simulink model "fuelCycle_w_trapping"  (R2023b)
settings: Solver=ode15s  StartTime=0.0  StopTime=sim_time  MinStep=1e-4  RelTol=1e-4
values from neighbouring files (symbols this model uses):
  AF = 90    [BOTH_scenario_inputData.m]    (also in FC_scenario_inputData.m; PO_scenario_inputData.m = 0.7; inputData.m = 70; parametric_analysis_AF.m = AF_array(i))
  eta2 = 0.95    [BOTH_scenario_inputData.m]    (also in FC_scenario_inputData.m; PO_scenario_inputData.m; inputData.m; parametric_analysis_eta_tes.m = eta_tes_array(i))
  f51 = 0.33    [BOTH_scenario_inputData.m]    (also in FC_scenario_inputData.m; PO_scenario_inputData.m; inputData.m; worst_case_InputData.m)
  f53 = 0.33    [BOTH_scenario_inputData.m]    (also in FC_scenario_inputData.m; PO_scenario_inputData.m; inputData.m; worst_case_InputData.m)
  f54 = 1 - f51 - f53 - f56    (= 0.3399)    [BOTH_scenario_inputData.m]    (also in FC_scenario_inputData.m; PO_scenario_inputData.m; inputData.m; worst_case_InputData.m)
  f96 = 0.1    [BOTH_scenario_inputData.m]    (also in FC_scenario_inputData.m; PO_scenario_inputData.m; inputData.m; worst_case_InputData.m)
  f_dir = 0.7    [BOTH_scenario_inputData.m]    (also in FC_scenario_inputData.m; PO_scenario_inputData.m = 0.3; inputData.m = 0.3; parametric_analysis_f_dir.m = f_dir_array(i))
  f_permanent_trap = 0    [inputData_trapping.m]    (also in parametric_analysis_trapping.m = f_permanent_trap_array(i))
  f_permanent_trap_structural = 0    [inputData_trapping.m]
  fp3 = 1e-4    (= 0.0001)    [BOTH_scenario_inputData.m]    (also in FC_scenario_inputData.m; PO_scenario_inputData.m; inputData.m; parametric_analysis_f_p.m = f_p(i) / 2)
  fp4 = 1e-4    (= 0.0001)    [BOTH_scenario_inputData.m]    (also in FC_scenario_inputData.m; PO_scenario_inputData.m; inputData.m; parametric_analysis_f_p.m = f_p(i) / 2)
  I_s_0 = 1.4    [fuelCycleSimulator.m]    (also in parametric_analysis_AF.m = 0.8; parametric_analysis_epsi.m = 0.8; parametric_analysis_eta_tes.m = 0.8; parametric_analysis_f_dir.m = 0.8)
  lambda = 1.73e-9    (= 1.73e-09)    [BOTH_scenario_inputData.m]    (also in FC_scenario_inputData.m; PO_scenario_inputData.m; inputData.m; inputData_trapping.m = a_tungsten/2/sqrt(2))
  m_u = 1.6e-27    [inputData_trapping-lap-meschini.m]    (also in inputData_trapping.m)
  N_dot = 8.99e-7    (= 8.99e-07)    [BOTH_scenario_inputData.m]    (also in FC_scenario_inputData.m = 9.3e-07; PO_scenario_inputData.m = 9.3e-07; inputData.m = 9.3e-07; worst_case_InputData.m = 9.3e-07)
  n_structural = (rho_structural*1e3) / PM_structural * N_a    (= 7.36894684052e+25)    [inputData_trapping-lap-meschini.m]    (also in inputData_trapping.m = 2.57913139418e+29)
  n_trap = 1e-4    (= 0.0001)    [inputData_trapping.m]    (also in parametric_analysis_trapping.m = n_trap_array(j))
  n_trap_structural = n_trap_vcrti    (= 0.0001)    [inputData_trapping-lap-meschini.m]    (also in inputData_trapping.m; parametric_analysis_trapping.m = n_trap_array(j))
  n_tungsten = (rho_tungsten*1e3) / PM_tungsten * N_a    (= 6.32342763874e+25)    [inputData_trapping-lap-meschini.m]    (also in inputData_trapping.m = 2.21319967356e+28)
  T1 = 1/((1 + epsi)/tau1 + lambda)    [BOTH_scenario_inputData.m]    (also in FC_scenario_inputData.m; PO_scenario_inputData.m; inputData.m; parametric_analysis_epsi.m)
  T12 = 1/((1 + epsi)/tau12 + lambda)    [BOTH_scenario_inputData.m]    (also in FC_scenario_inputData.m; PO_scenario_inputData.m; inputData.m; parametric_analysis_epsi.m)
  T2 = 1/((1 + epsi)/tau2 + lambda)    [BOTH_scenario_inputData.m]    (also in FC_scenario_inputData.m; PO_scenario_inputData.m; inputData.m; parametric_analysis_epsi.m)
  T3 = 1/((1 + 0)/tau3 + lambda)    [BOTH_scenario_inputData.m]    (also in FC_scenario_inputData.m; PO_scenario_inputData.m; inputData.m; parametric_analysis_epsi.m)
  T4 = 1/((1 + 0)/tau4 + lambda)    [BOTH_scenario_inputData.m]    (also in FC_scenario_inputData.m; PO_scenario_inputData.m; inputData.m; parametric_analysis_epsi.m)
  T7 = 1/((1 + epsi)/tau7 + lambda)    [BOTH_scenario_inputData.m]    (also in FC_scenario_inputData.m; PO_scenario_inputData.m; inputData.m; parametric_analysis_epsi.m)
  T8 = 1/((1 + epsi)/tau8 + lambda)    [BOTH_scenario_inputData.m]    (also in FC_scenario_inputData.m; PO_scenario_inputData.m; inputData.m; parametric_analysis_TBE.m)
  T9 = 1/((1 + epsi)/tau9 + lambda)    [BOTH_scenario_inputData.m]    (also in FC_scenario_inputData.m; PO_scenario_inputData.m; inputData.m; parametric_analysis_TBE.m)
  T_replacement = 100*8760*3600    (= 3153600000)    [inputData.m]
  tau1 = 1.25*3600    (= 4500)    [BOTH_scenario_inputData.m]    (also in FC_scenario_inputData.m; PO_scenario_inputData.m; inputData.m; parametric_analysis_t_blanket.m = tau1_array(i))
  tau12 = 100    [BOTH_scenario_inputData.m]    (also in FC_scenario_inputData.m; PO_scenario_inputData.m; inputData.m; worst_case_InputData.m)
  tau2 = 1*24*3600    (= 86400)    [BOTH_scenario_inputData.m]    (also in FC_scenario_inputData.m; PO_scenario_inputData.m; inputData.m; worst_case_InputData.m)
  tau3 = 1000    [BOTH_scenario_inputData.m]    (also in FC_scenario_inputData.m; PO_scenario_inputData.m; inputData.m; worst_case_InputData.m)
  tau4 = 1000    [BOTH_scenario_inputData.m]    (also in FC_scenario_inputData.m; PO_scenario_inputData.m; inputData.m; worst_case_InputData.m)
  tau5 = 1000    [BOTH_scenario_inputData.m]    (also in FC_scenario_inputData.m; PO_scenario_inputData.m; inputData.m; worst_case_InputData.m)
  tau6 = 3600    [BOTH_scenario_inputData.m]    (also in FC_scenario_inputData.m; PO_scenario_inputData.m; inputData.m; worst_case_InputData.m)
  tau7 = 600    [BOTH_scenario_inputData.m]    (also in FC_scenario_inputData.m; PO_scenario_inputData.m; inputData.m; worst_case_InputData.m)
  tau8 = 0.1*3600    (= 360)    [BOTH_scenario_inputData.m]    (also in FC_scenario_inputData.m; PO_scenario_inputData.m; inputData.m = 3600; parametric_analysis_TBE.m = t_p*0.1)
  tau9 = 0.9*3600    (= 3240)    [BOTH_scenario_inputData.m]    (also in FC_scenario_inputData.m; PO_scenario_inputData.m = 14040; inputData.m = 10800; parametric_analysis_TBE.m = t_p*0.9)
  tau_detrap = 1 / nu_detrap* relaxation_coefficient    [inputData_trapping.m]
  tau_detrap_structural = 1 / nu_detrap_structural* relaxation_coefficient    [inputData_trapping-lap-meschini.m]    (also in inputData_trapping.m)
  tau_permanent = 100 * 24 *3600    (= 8640000)    [inputData_trapping.m]
  tau_permanent_structural = 100 * 24 *3600    (= 8640000)    [inputData_trapping.m]
  TBE = 0.1    [BOTH_scenario_inputData.m]    (also in FC_scenario_inputData.m = 0.02; PO_scenario_inputData.m; inputData.m = 0.02; parametric_analysis_AF.m = TBE_array(j))
  TBR = 1.06    [fuelCycleSimulator.m]    (also in parametric_analysis_AF.m = 1; parametric_analysis_TBE.m = 1; parametric_analysis_epsi.m = 1; parametric_analysis_eta_tes.m = 1)
  V_structural = 3.5e6    (= 3500000)    [inputData_trapping-lap-meschini.m]    (also in inputData_trapping.m)
  V_tungsten = 0.35e6    (= 350000)    [inputData_trapping-lap-meschini.m]    (also in inputData_trapping.m)
libraries: arc x4
settings Model: SimulationMode=accelerator  Creator=smesc  LastModifiedBy=smesc
settings SolverCC: InitialStep=1e-4  MaxConsecutiveMinStep=10  ShapePreserveControl=EnableAll  ZeroCrossAlgorithm=Adaptive
settings OptimizationCC: ReuseModelBlockBuffer=off
settings ModelReferenceCC: EnableRefExpFcnMdlSchedulingChecks=on

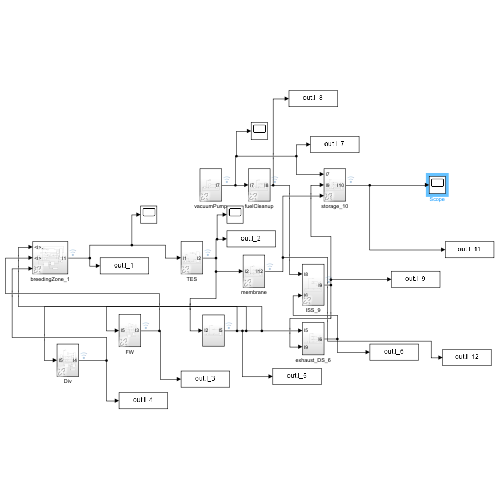
[thumbnail: Simulink's stored preview of the top-level diagram]
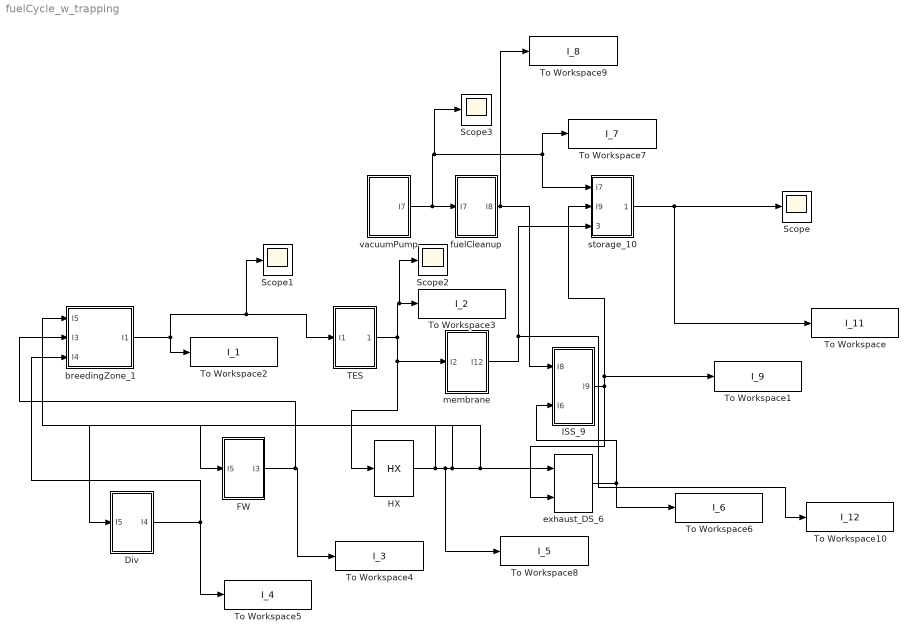
== system fuelCycle_w_trapping ==
  Div : Subsystem  AncestorBlock=arc/divertor_4
      settings: LibrarySourceBlock=arc/divertor_4
  FW : Subsystem  AncestorBlock=arc/FW_3
      settings: LibrarySourceBlock=arc/FW_3
  HX : arc/HX  Tag=HX  SystemSampleTime=-1  VariantActivationTime=update diagram  AllowFlexibleInterface=on  Latency=0  AutoFrameSizeCalculation=off
  ISS_9 : Subsystem  AncestorBlock=arc/ISS_9
      settings: LibrarySourceBlock=arc/ISS_9
  Scope{,1..3} (4 alike) : Scope
  TES : Subsystem  AncestorBlock=arc/TES_2
      settings: LibrarySourceBlock=arc/TES_2
  To Workspace : ToWorkspace  VariableName=I_11  SampleTime=-1
  To Workspace1 : ToWorkspace  VariableName=I_9  SampleTime=-1
  To Workspace10 : ToWorkspace  VariableName=I_12  SampleTime=-1
  To Workspace2 : ToWorkspace  VariableName=I_1  SampleTime=-1
  To Workspace3 : ToWorkspace  VariableName=I_2  SampleTime=-1
  To Workspace4 : ToWorkspace  VariableName=I_3  SampleTime=-1
  To Workspace5 : ToWorkspace  VariableName=I_4  SampleTime=-1
  To Workspace6 : ToWorkspace  VariableName=I_6  SampleTime=-1
  To Workspace7 : ToWorkspace  VariableName=I_7  SampleTime=-1
  To Workspace8 : ToWorkspace  VariableName=I_5  SampleTime=-1
  To Workspace9 : ToWorkspace  VariableName=I_8  SampleTime=-1
  breedingZone_1 : Subsystem  AncestorBlock=arc/breedingZone_1
      settings: LibrarySourceBlock=arc/breedingZone_1
  exhaust_DS_6 : arc/exhaust_DS  SystemSampleTime=-1  VariantActivationTime=update diagram  AllowFlexibleInterface=on  Latency=0  AutoFrameSizeCalculation=off
      link override Gain: Gain=f56/tau5
  fuelCleanup : Subsystem  AncestorBlock=arc/fuelCleanUp
  membrane : Subsystem  AncestorBlock=arc/fuelCleanUp_8
      settings: LibrarySourceBlock=arc/fuelCleanUp_8
  storage_10 : Subsystem  AncestorBlock=arc/storage_10
      settings: LibrarySourceBlock=arc/storage_10
  vacuumPump : Subsystem  AncestorBlock=arc/pump_7
      settings: LibrarySourceBlock=arc/pump_7
  wires:
  breedingZone_1/1(I1) -> Scope1/1, TES/1(I1), To Workspace2/1
  storage_10/1(I10) -> To Workspace/1, Scope/1
  FW/1(I3) -> breedingZone_1/2(I3), To Workspace4/1
  Div/1(I4) -> breedingZone_1/3(I4), To Workspace5/1
  membrane/1(I12) -> To Workspace10/1, storage_10/3(I12)
  fuelCleanup/1(I8) -> To Workspace9/1, ISS_9/1(I8)
  vacuumPump/1(I7) -> Scope3/1, To Workspace7/1, storage_10/1(I7), fuelCleanup/1(I7)
  exhaust_DS_6/1 -> ISS_9/2(I6), To Workspace6/1
  ISS_9/1(I9) -> exhaust_DS_6/2, storage_10/2(I9), To Workspace1/1
  HX/1 -> FW/1(I5), To Workspace8/1, Div/1(I5), exhaust_DS_6/1, breedingZone_1/1(I5)
  TES/1(Output) -> Scope2/1, To Workspace3/1, membrane/1(I2), HX/1

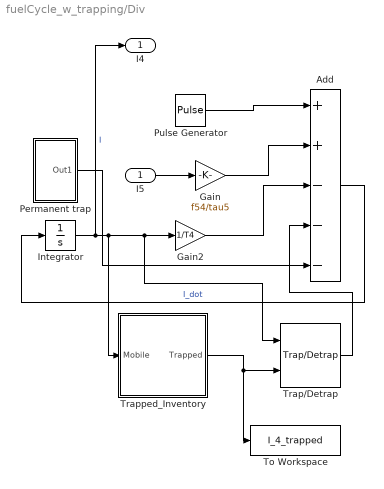
== system fuelCycle_w_trapping/Div ==
  I5 : Inport
  Add : Sum  Inputs=++---
  Gain : Gain  Gain=f54/tau5
  Gain2 : Gain  Gain=1/T4
  Integrator : Integrator
  Permanent trap : Subsystem
  Pulse Generator : DiscretePulseGenerator  PulseType=Time based  Amplitude=fp4*N_dot/TBE  Period=1800  PulseWidth=AF
  To Workspace : ToWorkspace  VariableName=I_4_trapped  SampleTime=-1
  Trap/Detrap : arc/Trap//Detrap  SystemSampleTime=-1  VariantActivationTime=update diagram  AllowFlexibleInterface=on  Latency=0  AutoFrameSizeCalculation=off
  Trapped_Inventory : Subsystem  AncestorBlock=arc/Trapped_Inventory
  I4 : Outport
  wires:
  Pulse Generator/1 -> Add/1
  Gain/1 -> Add/2
  Integrator/1 -> Trapped_Inventory/1(Mobile), Trap/Detrap/1, Gain2/1, I4/1  "I"
  Add/1 -> Integrator/1  "I_dot"
  Gain2/1 -> Add/3
  I5/1 -> Gain/1
  Trapped_Inventory/1(Trapped) -> To Workspace/1, Trap/Detrap/2
  Trap/Detrap/1 -> Add/4
  Permanent trap/1(Out1) -> Add/5

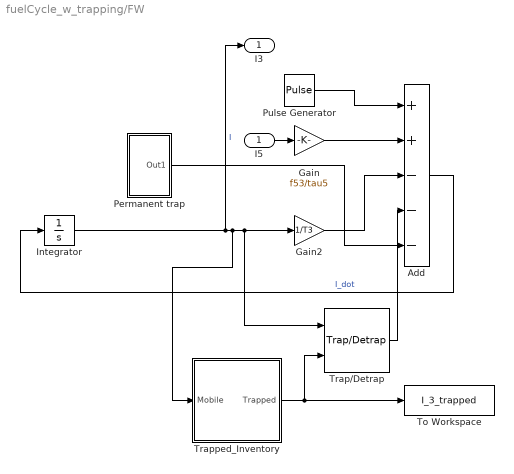
== system fuelCycle_w_trapping/FW ==
  I5 : Inport
  Add : Sum  Inputs=++---
  Gain : Gain  Gain=f53/tau5
  Gain2 : Gain  Gain=1/T3
  Integrator : Integrator
  Permanent trap : Subsystem
  Pulse Generator : DiscretePulseGenerator  PulseType=Time based  Amplitude=fp3*N_dot/TBE  Period=1800  PulseWidth=AF
  To Workspace : ToWorkspace  VariableName=I_3_trapped  SampleTime=-1
  Trap/Detrap : arc/Trap//Detrap  SystemSampleTime=-1  VariantActivationTime=update diagram  AllowFlexibleInterface=on  Latency=0  AutoFrameSizeCalculation=off
  Trapped_Inventory : Subsystem  AncestorBlock=arc/Trapped_Inventory
  I3 : Outport
  wires:
  Gain2/1 -> Add/3
  Pulse Generator/1 -> Add/1
  Integrator/1 -> I3/1, Trapped_Inventory/1(Mobile), Trap/Detrap/1, Gain2/1  "I"
  Add/1 -> Integrator/1  "I_dot"
  Gain/1 -> Add/2
  I5/1 -> Gain/1
  Trap/Detrap/1 -> Add/4
  Trapped_Inventory/1(Trapped) -> Trap/Detrap/2, To Workspace/1
  Permanent trap/1(Out1) -> Add/5

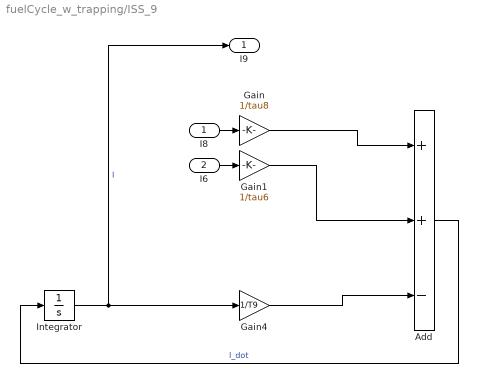
== system fuelCycle_w_trapping/ISS_9 ==
  I8 : Inport
  I6 : Inport  Port=2
  Add : Sum  Inputs=++-
  Gain : Gain  Gain=1/tau8
  Gain1 : Gain  Gain=1/tau6
  Gain4 : Gain  Gain=1/T9
  Integrator : Integrator
  I9 : Outport
  wires:
  I8/1 -> Gain/1
  Gain1/1 -> Add/2
  I6/1 -> Gain1/1
  Add/1 -> Integrator/1  "I_dot"
  Integrator/1 -> Gain4/1, I9/1  "I"
  Gain/1 -> Add/1
  Gain4/1 -> Add/3

== system fuelCycle_w_trapping/TES ==
  I1 : Inport
  Add : Sum  Inputs=+-
  Gain : Gain  Gain=1/T2
  Gain1 : Gain  Gain=1/tau1
  Integrator : Integrator
  Output : Outport
  wires:
  Gain/1 -> Add/2
  I1/1 -> Gain1/1
  Gain1/1 -> Add/1
  Integrator/1 -> Gain/1, Output/1  "I2"
  Add/1 -> Integrator/1  "I_dot"

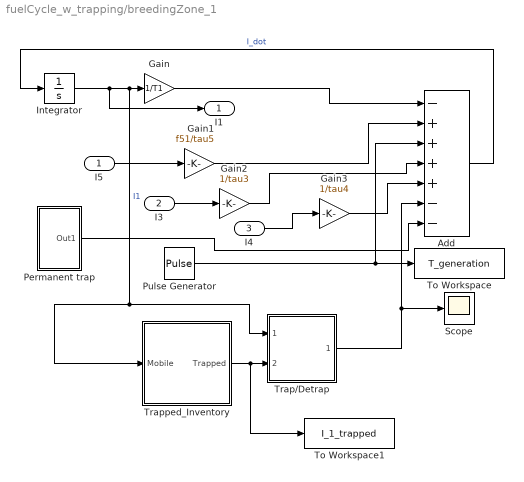
== system fuelCycle_w_trapping/breedingZone_1 ==
  I5 : Inport
  I3 : Inport  Port=2
  I4 : Inport  Port=3
  Add : Sum  Inputs=-++++--
  Gain : Gain  Gain=1/T1
  Gain1 : Gain  Gain=f51/tau5
  Gain2 : Gain  Gain=1/tau3
  Gain3 : Gain  Gain=1/tau4
  Integrator : Integrator
  Permanent trap : Subsystem
  Pulse Generator : DiscretePulseGenerator  PulseType=Time based  Amplitude=N_dot * TBR  Period=1800  PulseWidth=AF
  Scope : Scope
  To Workspace : ToWorkspace  VariableName=T_generation  SaveFormat=Timeseries  SampleTime=-1
  To Workspace1 : ToWorkspace  VariableName=I_1_trapped  SampleTime=-1
  Trap/Detrap : Subsystem  AncestorBlock=arc/Trap//Detrap
  Trapped_Inventory : Subsystem  AncestorBlock=arc/Trapped_Inventory
  I1 : Outport
  wires:
  Add/1 -> Integrator/1  "I_dot"
  Gain1/1 -> Add/2
  Integrator/1 -> Trapped_Inventory/1(Mobile), Trap/Detrap/1(Mobile), Gain/1, I1/1  "I1"
  Gain/1 -> Add/1
  I5/1 -> Gain1/1
  Pulse Generator/1 -> Add/3, To Workspace/1
  I3/1 -> Gain2/1
  Gain2/1 -> Add/4
  I4/1 -> Gain3/1
  Gain3/1 -> Add/5
  Trapped_Inventory/1(Trapped) -> To Workspace1/1, Trap/Detrap/2(Trapped)
  Trap/Detrap/1(trap_detrap) -> Scope/1, Add/6
  Permanent trap/1(Out1) -> Add/7

== system fuelCycle_w_trapping/fuelCleanup ==
  I7 : Inport
  Add : Sum  Inputs=+-
  Gain : Gain  Gain=(1-f_dir)/tau7
  Gain1 : Gain  Gain=1/T8
  Integrator : Integrator
  I8 : Outport
  wires:
  I7/1 -> Gain/1
  Gain1/1 -> Add/2
  Add/1 -> Integrator/1  "I_dot"
  Integrator/1 -> Gain1/1, I8/1  "I"
  Gain/1 -> Add/1

== system fuelCycle_w_trapping/membrane ==
  I2 : Inport
  Add : Sum  Inputs=+-
  Gain : Gain  Gain=eta2/tau2
  Gain1 : Gain  Gain=1/T12
  Integrator : Integrator
  I12 : Outport
  wires:
  I2/1 -> Gain/1
  Gain1/1 -> Add/2
  Add/1 -> Integrator/1  "I_dot"
  Integrator/1 -> Gain1/1, I12/1  "I"
  Gain/1 -> Add/1

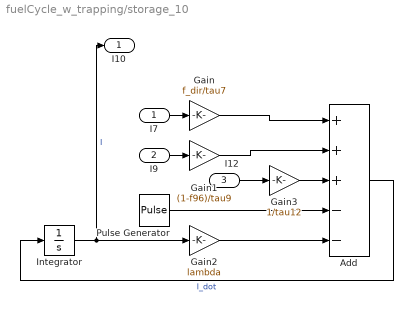
== system fuelCycle_w_trapping/storage_10 ==
  I7 : Inport
  I9 : Inport  Port=2
  I12 : Inport  Port=3
  Add : Sum  Inputs=+++--
  Gain : Gain  Gain=f_dir/tau7
  Gain1 : Gain  Gain=(1-f96)/tau9
  Gain2 : Gain  Gain=lambda
  Gain3 : Gain  Gain=1/tau12
  Integrator : Integrator  InitialCondition=I_s_0
  Pulse Generator : DiscretePulseGenerator  PulseType=Time based  Amplitude=N_dot/TBE  Period=1800  PulseWidth=AF
  I10 : Outport
  wires:
  Integrator/1 -> Gain2/1, I10/1  "I"
  I9/1 -> Gain1/1
  Gain2/1 -> Add/5
  I7/1 -> Gain/1
  Gain1/1 -> Add/2
  Gain/1 -> Add/1
  Pulse Generator/1 -> Add/4
  I12/1 -> Gain3/1
  Gain3/1 -> Add/3
  Add/1 -> Integrator/1  "I_dot"

== system fuelCycle_w_trapping/vacuumPump ==
  Add : Sum  Inputs=+-
  Gain : Gain  Gain=1/T7
  Integrator : Integrator
  Pulse Generator : DiscretePulseGenerator  PulseType=Time based  Amplitude=(1-TBE-fp3-fp4)*N_dot/TBE  Period=1800  PulseWidth=AF
  I7 : Outport
  wires:
  Gain/1 -> Add/2
  Integrator/1 -> Gain/1, I7/1  "I7"
  Pulse Generator/1 -> Add/1
  Add/1 -> Integrator/1  "I_dot"

== system fuelCycle_w_trapping/Div/Permanent trap ==
  Clock : Clock
  Exp : Math
  Gain1 : Gain  Gain=-1/tau_permanent
  Gain3 : Gain  Gain=f_permanent_trap*n_trap*n_tungsten*3*m_u*1*(V_tungsten/2)
  Scope : Scope
  Out1 : Outport
  wires:
  Gain3/1 -> Scope/1, Out1/1
  Clock/1 -> Gain1/1
  Gain1/1 -> Exp/1
  Exp/1 -> Gain3/1

== system fuelCycle_w_trapping/Div/Trapped_Inventory ==
  Mobile : Inport
  Integrator1 : Integrator
  Trap/Detrap : Subsystem
  Trapped : Outport
  wires:
  Trap/Detrap/1(Out1) -> Integrator1/1
  Mobile/1 -> Trap/Detrap/1(In1)
  Integrator1/1 -> Trap/Detrap/2(In2), Trapped/1

== system fuelCycle_w_trapping/FW/Permanent trap ==
  Clock : Clock
  Exp : Math
  Gain1 : Gain  Gain=-1/tau_permanent
  Gain3 : Gain  Gain=f_permanent_trap*n_trap*n_tungsten*3*m_u*1*(V_tungsten/2)
  Scope : Scope
  Out1 : Outport
  wires:
  Gain3/1 -> Scope/1, Out1/1
  Clock/1 -> Gain1/1
  Gain1/1 -> Exp/1
  Exp/1 -> Gain3/1

== system fuelCycle_w_trapping/FW/Trapped_Inventory ==
  Mobile : Inport
  Integrator1 : Integrator
  Trap/Detrap : Subsystem
  Trapped : Outport
  wires:
  Trap/Detrap/1(Out1) -> Integrator1/1
  Mobile/1 -> Trap/Detrap/1(In1)
  Integrator1/1 -> Trap/Detrap/2(In2), Trapped/1

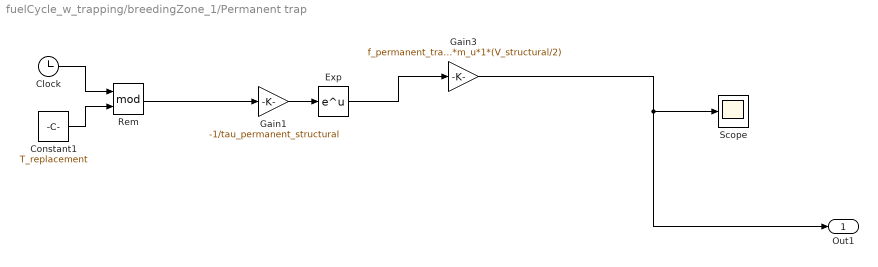
== system fuelCycle_w_trapping/breedingZone_1/Permanent trap ==
  Clock : Clock
  Constant1 : Constant  Value=T_replacement
  Exp : Math
  Gain1 : Gain  Gain=-1/tau_permanent_structural
  Gain3 : Gain  Gain=f_permanent_trap_structural*n_trap_structural*n_structural*3*m_u*1*(V_structural/2)
  Rem : Math  Operator=mod
  Scope : Scope
  Out1 : Outport
  wires:
  Gain3/1 -> Scope/1, Out1/1
  Gain1/1 -> Exp/1
  Exp/1 -> Gain3/1
  Clock/1 -> Rem/1
  Constant1/1 -> Rem/2
  Rem/1 -> Gain1/1

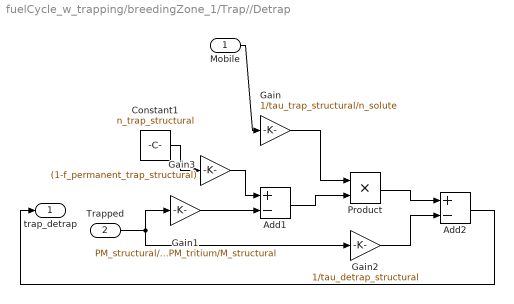
== system fuelCycle_w_trapping/breedingZone_1/Trap//Detrap ==
  Mobile : Inport
  Trapped : Inport  Port=2
  Add1 : Sum  Inputs=+-
  Add2 : Sum  Inputs=+-
  Constant1 : Constant  Value=n_trap_structural
  Gain : Gain  Gain=1/tau_trap_structural/n_solute
  Gain1 : Gain  Gain=PM_structural/PM_tritium/M_structural
  Gain2 : Gain  Gain=1/tau_detrap_structural
  Gain3 : Gain  Gain=(1-f_permanent_trap_structural)
  Product : Product
  trap_detrap : Outport
  wires:
  Trapped/1 -> Gain1/1, Gain2/1
  Gain1/1 -> Add1/2
  Add1/1 -> Product/2
  Gain2/1 -> Add2/2
  Gain/1 -> Product/1
  Mobile/1 -> Gain/1
  Add2/1 -> trap_detrap/1
  Product/1 -> Add2/1
  Constant1/1 -> Gain3/1
  Gain3/1 -> Add1/1

== system fuelCycle_w_trapping/breedingZone_1/Trapped_Inventory ==
  Mobile : Inport
  Clock : Clock
  Constant1 : Constant  Value=T_replacement
  Integrator1 : Integrator  ExternalReset=falling
  Rem : Math  Operator=mod
  Trap/Detrap : Subsystem
  Trapped : Outport
  wires:
  Trap/Detrap/1(Out1) -> Integrator1/1
  Mobile/1 -> Trap/Detrap/1(In1)
  Integrator1/1 -> Trap/Detrap/2(In2), Trapped/1
  Clock/1 -> Rem/1
  Rem/1 -> Integrator1/2
  Constant1/1 -> Rem/2

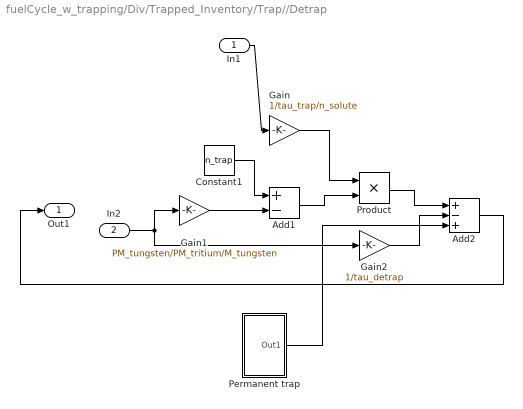
== system fuelCycle_w_trapping/Div/Trapped_Inventory/Trap//Detrap ==
  In1 : Inport
  In2 : Inport  Port=2
  Add1 : Sum  Inputs=+-
  Add2 : Sum  Inputs=+-+
  Constant1 : Constant  Value=n_trap
  Gain : Gain  Gain=1/tau_trap/n_solute
  Gain1 : Gain  Gain=PM_tungsten/PM_tritium/M_tungsten
  Gain2 : Gain  Gain=1/tau_detrap
  Permanent trap : Subsystem
  Product : Product
  Out1 : Outport
  wires:
  In2/1 -> Gain1/1, Gain2/1
  Gain1/1 -> Add1/2
  Add1/1 -> Product/2
  Gain2/1 -> Add2/2
  Constant1/1 -> Add1/1
  Gain/1 -> Product/1
  In1/1 -> Gain/1
  Add2/1 -> Out1/1
  Product/1 -> Add2/1
  Permanent trap/1(Out1) -> Add2/3

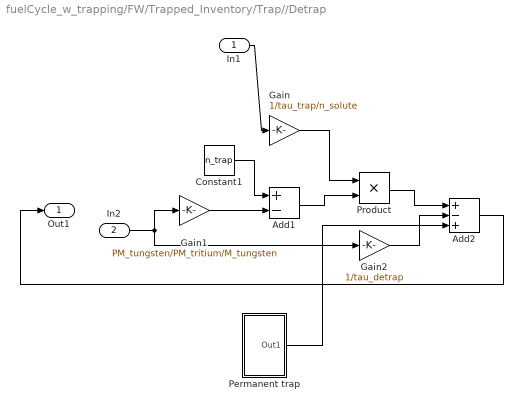
== system fuelCycle_w_trapping/FW/Trapped_Inventory/Trap//Detrap ==
  In1 : Inport
  In2 : Inport  Port=2
  Add1 : Sum  Inputs=+-
  Add2 : Sum  Inputs=+-+
  Constant1 : Constant  Value=n_trap
  Gain : Gain  Gain=1/tau_trap/n_solute
  Gain1 : Gain  Gain=PM_tungsten/PM_tritium/M_tungsten
  Gain2 : Gain  Gain=1/tau_detrap
  Permanent trap : Subsystem
  Product : Product
  Out1 : Outport
  wires:
  In2/1 -> Gain1/1, Gain2/1
  Gain1/1 -> Add1/2
  Add1/1 -> Product/2
  Gain2/1 -> Add2/2
  Constant1/1 -> Add1/1
  Gain/1 -> Product/1
  In1/1 -> Gain/1
  Add2/1 -> Out1/1
  Product/1 -> Add2/1
  Permanent trap/1(Out1) -> Add2/3

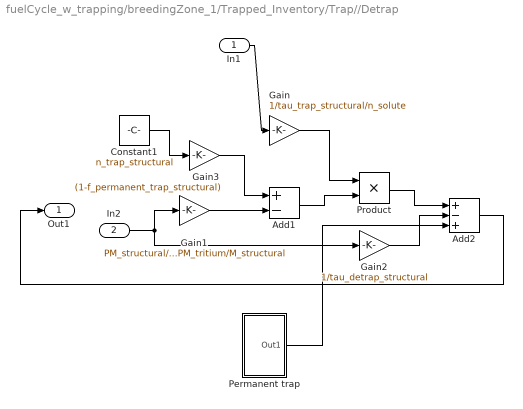
== system fuelCycle_w_trapping/breedingZone_1/Trapped_Inventory/Trap//Detrap ==
  In1 : Inport
  In2 : Inport  Port=2
  Add1 : Sum  Inputs=+-
  Add2 : Sum  Inputs=+-+
  Constant1 : Constant  Value=n_trap_structural
  Gain : Gain  Gain=1/tau_trap_structural/n_solute
  Gain1 : Gain  Gain=PM_structural/PM_tritium/M_structural
  Gain2 : Gain  Gain=1/tau_detrap_structural
  Gain3 : Gain  Gain=(1-f_permanent_trap_structural)
  Permanent trap : Subsystem
  Product : Product
  Out1 : Outport
  wires:
  In2/1 -> Gain1/1, Gain2/1
  Gain1/1 -> Add1/2
  Add1/1 -> Product/2
  Gain2/1 -> Add2/2
  Gain/1 -> Product/1
  In1/1 -> Gain/1
  Add2/1 -> Out1/1
  Product/1 -> Add2/1
  Permanent trap/1(Out1) -> Add2/3
  Constant1/1 -> Gain3/1
  Gain3/1 -> Add1/1

== system fuelCycle_w_trapping/Div/Trapped_Inventory/Trap//Detrap/Permanent trap ==
  Clock : Clock
  Exp : Math
  Gain1 : Gain  Gain=-1/tau_permanent
  Gain3 : Gain  Gain=f_permanent_trap*n_trap*n_tungsten*3*m_u*1*(V_tungsten/2)
  Scope : Scope
  Out1 : Outport
  wires:
  Gain3/1 -> Scope/1, Out1/1
  Clock/1 -> Gain1/1
  Gain1/1 -> Exp/1
  Exp/1 -> Gain3/1

== system fuelCycle_w_trapping/FW/Trapped_Inventory/Trap//Detrap/Permanent trap ==
  Clock : Clock
  Exp : Math
  Gain1 : Gain  Gain=-1/tau_permanent
  Gain3 : Gain  Gain=f_permanent_trap*n_trap*n_tungsten*3*m_u*1*(V_tungsten/2)
  Scope : Scope
  Out1 : Outport
  wires:
  Gain3/1 -> Scope/1, Out1/1
  Clock/1 -> Gain1/1
  Gain1/1 -> Exp/1
  Exp/1 -> Gain3/1

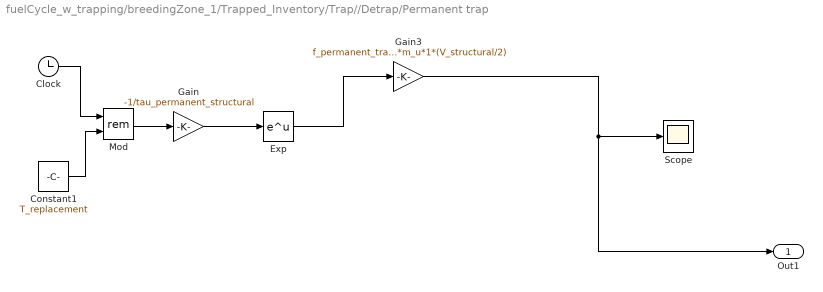
== system fuelCycle_w_trapping/breedingZone_1/Trapped_Inventory/Trap//Detrap/Permanent trap ==
  Clock : Clock
  Constant1 : Constant  Value=T_replacement
  Exp : Math
  Gain : Gain  Gain=-1/tau_permanent_structural
  Gain3 : Gain  Gain=f_permanent_trap_structural*n_trap_structural*n_structural*3*m_u*1*(V_structural/2)
  Mod : Math  Operator=rem
  Scope : Scope
  Out1 : Outport
  wires:
  Gain3/1 -> Scope/1, Out1/1
  Exp/1 -> Gain3/1
  Constant1/1 -> Mod/2
  Clock/1 -> Mod/1
  Gain/1 -> Exp/1
  Mod/1 -> Gain/1
